simulink model "motor_sim"  (Simulink 7.1)
settings: Solver=FixedStepDiscrete  StartTime=0.0  StopTime=60  FixedStep=0.1  RelTol=1e-3
libraries: arduino_io_lib x3, simulink x1
settings Model: Creator=gcampa  LastModifiedBy=gcampa
settings OptimizationCC: InitFltsAndDblsToZero=off
settings DebuggingCC: StrictBusMsg=ErrorLevel1
settings GRTTargetCC: CPPClassGenCompliant=off

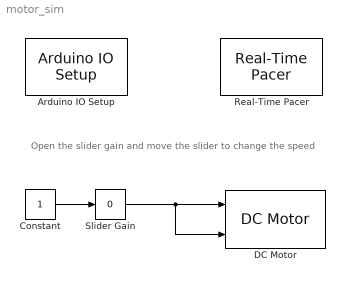
== system motor_sim ==
  note: Open the slider gain and move the slider to change the speed
  Arduino IO Setup : arduino_io_lib/Arduino IO Setup  Priority=3  arduinoVar=Arduino1  comPort=COM9
  Constant : Constant
  DC Motor : arduino_io_lib/DC Motor  arduinoVar=Arduino1  motorNum=4  sendOnChange=on  T=0.2
  Real-Time Pacer : arduino_io_lib/Real-Time Pacer  simTimePerRealTime=1
  Slider Gain : simulink/Math Operations/Slider Gain  SystemSampleTime=-1  low=-255  gain=0  high=255
  wires:
  Constant/1 -> Slider Gain/1
  Slider Gain/1 -> DC Motor/1, DC Motor/2
